simulink model "Friction_Estimation"  (R2024b)
settings: Solver=VariableStepAuto  StartTime=0.0  StopTime=45  RelTol=1e-3
InitFcn:
  | Init
values from neighbouring files (symbols this model uses):
  degs2rpm = 60/360    (= 0.166666666667)    [Init.m]    (also in ModelParams.m; load_params_inertial_case.m)
  delta_est = 1/sqrt(2)    [Init.m]    (also in code.m; main.m)
  Kd = Kp * Td    [Init.m]    (also in code.m; main.m)
  Ki = Kp / Ti    [Init.m]    (also in code.m; main.m)
  Kp = deltak * cos(deltaphi)    [Init.m]    (also in code.m = deltak*cos(deltaphi); main.m = deltak*cos(deltaphi))
  rpm2degs = 360/60    (= 6)    [Init.m]    (also in ModelParams.m; load_params_inertial_case.m)
  rpm2rads = 2*pi/60    (= 0.10471975512)    [Init.m]    (also in ModelParams.m; load_params_inertial_case.m)
  tl = 1/(3*wgc)    [Init.m]    (also in code.m = 1/cut_off; main.m = 1/cut_off)
  wc = 2*pi*20    (= 125.663706144)    [Init.m]    (also in code.m; main.m)
undefined symbols (not defined in the file or in its folder): gbox, mot, sens
libraries: simulink x2, SignalEditorBlockLib x1
settings Model: Creator=UTENTE041019  LastModifiedBy=lucag

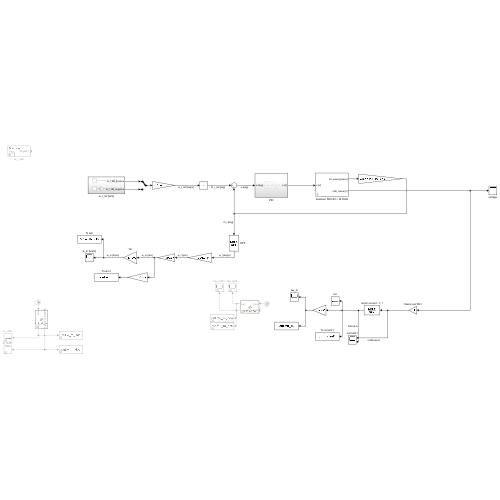
[thumbnail: Simulink's stored preview of the top-level diagram]
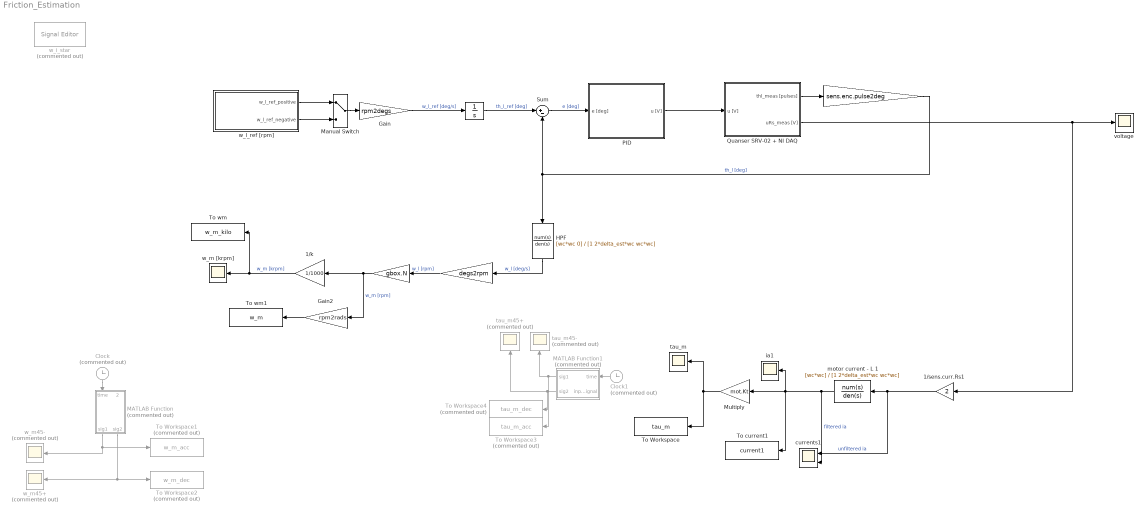
== system Friction_Estimation ==
  " " : Integrator
  "  " : Gain  Gain=sens.enc.pulse2deg
  "       " : Gain  Gain=degs2rpm
  "                  " : Gain  Gain=gbox.N
  1/k : Gain  Gain=1/1000
  1/sens.curr.Rs1 : Gain  Gain=2
  Clock : Clock  Commented=on
  Clock1 : Clock  Commented=on
  Gain : Gain  Gain=rpm2degs
  Gain2 : Gain  Gain=rpm2rads
  HPF : TransferFcn  Numerator=[wc*wc 0]  Denominator=[1 2*delta_est*wc wc*wc]
  MATLAB Function : MATLAB Function  Commented=on  TreatAsAtomicUnit=on
  MATLAB Function1 : MATLAB Function  Commented=on  TreatAsAtomicUnit=on
  Manual Switch : ManualSwitch
  Multiply : Gain  Gain=mot.Kt
  PID : Subsystem
  Quanser SRV-02 + NI DAQ : Subsystem  mask(Quanser SRV-02 (with inertial load) + NI DAQ){Ts=0.001, fricType=Coulomb + viscous}
      mask prompts: Ts "NI DAQ Sample Time:"; fricType "Friction model"
      mask help: Quanser SRV-02 (with inertial load) + NI DAQ model.
      mask init:
      | %%  Sensors data
      | 
      | %   shunt resistor
      | sens.curr.Rs = 0.5;                         %   resistance [Ohm]   
      | sens.curr.uRs_std = 0.01;                   %   voltage noise standard dev [V]                           
      | sens.curr.uRs_var = sens.curr.uRs_std^2;	%   voltage noise variance [V^2]
      | 
      | %   Hewlett-Packard HEDS-5540#A06 optical encoder
      | sens.enc.ppr = 500*4;                       %   pulses per rotation
      | sens.enc.pulse2deg = 360/sens.enc.ppr;      %   [pulses] -> [deg]
      | sens.enc.pulse2rad = 2*pi/sens.enc.ppr;     %   [pulses] -> [rad]
      | sens.enc.deg2pulse = sens.enc.ppr/360;      %   [deg] -> [pulses]
      | sens.enc.rad2pulse = sens.enc.ppr/2/pi;     %   [rad] -> [pulses]
      | 
      | 
      | %%  Data acquisition board (daq) data
      | 
      | %   NI PCI-6221 DAC data
      | daq.dac.bits = 16;                                  %   resolution (bits)
      | daq.dac.fs   = 10;                                  %   full scale 
      | daq.dac.q    = 2*daq.dac.fs/(2^daq.dac.bits-1);     %	quantization
      | 
      | %   NI PCI-6221 ADC data
      | daq.adc.bits = 16;                                  %   resolution (bits)
      | daq.adc.fs   = 10;                                  %   full scale (as set in SLDRT Analog Input block)
      | daq.adc.q    = 2*daq.adc.fs/(2^daq.adc.bits-1);     %   quantization
      mask Help:
      | Riccardo Antonello (antonello@dei.unipd.it)
      | 
      | April 24, 2020
      | 
      | Dept. of Information Engineering, University of Padova
      mask TypeOptions fricType: Coulomb + viscous | Karnopp
  Sum : Sum  Inputs=|+-
  To Workspace : ToWorkspace  VariableName=tau_m  SaveFormat=Structure With Time  SampleTime=-1
  To Workspace1 : ToWorkspace  Commented=on  VariableName=w_m_acc  SaveFormat=Structure With Time  SampleTime=-1
  To Workspace2 : ToWorkspace  Commented=on  VariableName=w_m_dec  SaveFormat=Structure With Time  SampleTime=-1
  To Workspace3 : ToWorkspace  Commented=on  VariableName=tau_m_acc  SaveFormat=Structure With Time  SampleTime=-1
  To Workspace4 : ToWorkspace  Commented=on  VariableName=tau_m_dec  SaveFormat=Structure With Time  SampleTime=-1
  To current1 : ToWorkspace  VariableName=current1  SaveFormat=Structure With Time  SampleTime=-1
  To wm : ToWorkspace  VariableName=w_m_kilo  SaveFormat=Structure With Time  SampleTime=-1
  To wm1 : ToWorkspace  VariableName=w_m  SaveFormat=Structure With Time  SampleTime=-1
  currents1 : Scope  NumInputPorts=2
  ia1 : Scope
  motor current - L 1 : TransferFcn  Numerator=[wc*wc]  Denominator=[1 2*delta_est*wc wc*wc]
  tau_m : Scope
  tau_m45+ : Scope  Commented=on
  tau_m45- : Scope  Commented=on
  voltage : Scope
  w_i_star : SignalEditorBlockLib/Signal Editor  Commented=on  FileName=untitled.mat  ActiveScenario=Scenario  ActiveSignal=Signal 1  IsBus=off  OutputBusObjectStr=Bus: BusObject  SampleTime=0  Interpolate=off  ZeroCross=off  OutputAfterFinalValue=Setting to zero  Unit=inherit  PreserveSignalName=on  ApplySigPropsToAllScenarios=on  ApplySigPropsToAllSignals=off
  w_l_ref [rpm] : Subsystem
  w_m [krpm] : Scope
  w_m45+ : Scope  Commented=on
  w_m45- : Scope  Commented=on
  wires:
  Sum/1 -> PID/1(e [deg])  "e [deg]"
  Quanser SRV-02 + NI DAQ/1(thl_meas [pulses]) -> "  "/1
  PID/1(u [V]) -> Quanser SRV-02 + NI DAQ/1(u [V])
  " "/1 -> Sum/1  "th_l_ref [deg]"
  "  "/1 -> HPF/1, Sum/2  "th_l [deg]"
  Quanser SRV-02 + NI DAQ/2(uRs_meas [V]) -> voltage/1, 1/sens.curr.Rs1/1
  1/sens.curr.Rs1/1 -> currents1/1, motor current - L 1/1  "unfiltered ia"
  motor current - L 1/1 -> currents1/2, ia1/1, Multiply/1, To current1/1  "filtered ia"
  HPF/1 -> "       "/1  "w_l [deg/s]"
  "       "/1 -> "                  "/1  "w_l [rpm]"
  "                  "/1 -> Gain2/1, 1/k/1  "w_m [rpm]"
  1/k/1 -> To wm/1, w_m [krpm]/1  "w_m [krpm]"
  Gain/1 -> " "/1  "w_l_ref [deg/s]"
  Clock/1 -> MATLAB Function/1(time)
  MATLAB Function/1(sig1) -> w_m45-/1, To Workspace1/1
  MATLAB Function/2(sig2) -> w_m45+/1, To Workspace2/1
  MATLAB Function1/2(sig2) -> tau_m45+/1, To Workspace4/1
  Clock1/1 -> MATLAB Function1/1(time)
  Multiply/1 -> tau_m/1, To Workspace/1
  MATLAB Function1/1(sig1) -> To Workspace3/1, tau_m45-/1
  w_l_ref [rpm]/1(w_l_ref_positive) -> Manual Switch/1
  w_l_ref [rpm]/2(w_l_ref_negative) -> Manual Switch/2
  Manual Switch/1 -> Gain/1
  Gain2/1 -> To wm1/1

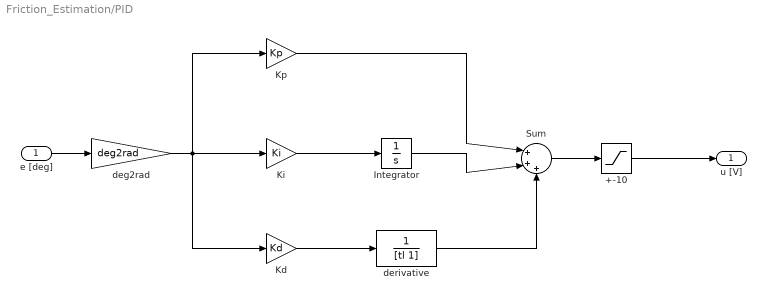
== system Friction_Estimation/PID ==
  e [deg] : Inport
  +-10 : Saturate  UpperLimit=10  LowerLimit=-10
  Integrator : Integrator
  Kd : Gain  Gain=Kd
  Ki : Gain  Gain=Ki
  Kp : Gain  Gain=Kp
  Sum : Sum  Inputs=|+++
  deg2rad : Gain  Gain=deg2rad
  derivative : TransferFcn  Denominator=[tl 1]
  u [V] : Outport
  wires:
  e [deg]/1 -> deg2rad/1
  deg2rad/1 -> Kd/1, Kp/1, Ki/1
  Ki/1 -> Integrator/1
  Kp/1 -> Sum/1
  Integrator/1 -> Sum/2
  Kd/1 -> derivative/1
  derivative/1 -> Sum/3
  Sum/1 -> +-10/1
  +-10/1 -> u [V]/1

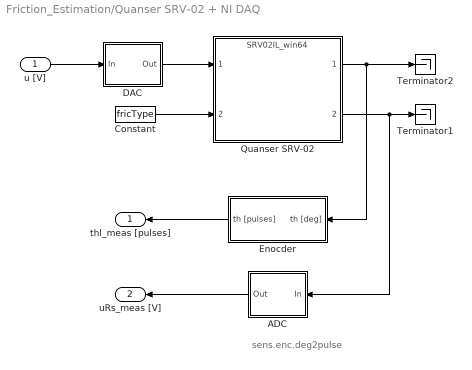
== system Friction_Estimation/Quanser SRV-02 + NI DAQ ==
  note: sens.enc.deg2pulse
  u [V] : Inport
  ADC : Subsystem
  Constant : Constant  Value=fricType
  DAC : Subsystem
  Enocder : Subsystem
  Quanser SRV-02 : ModelReference  ModelNameDialog=SRV02IL_win64.slxp  ModelReferenceVersion=1.44  CopyOfModelProtected=on
  Terminator1 : Terminator
  Terminator2 : Terminator
  thl_meas [pulses] : Outport
  uRs_meas [V] : Outport  Port=2
  wires:
  Enocder/1(th [pulses]) -> thl_meas [pulses]/1
  ADC/1(Out) -> uRs_meas [V]/1
  DAC/1(Out) -> Quanser SRV-02/1
  Quanser SRV-02/2 -> ADC/1(In), Terminator1/1
  u [V]/1 -> DAC/1(In)
  Quanser SRV-02/1 -> Enocder/1(th [deg]), Terminator2/1
  Constant/1 -> Quanser SRV-02/2

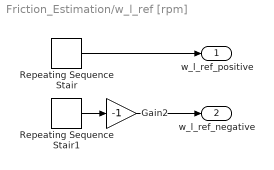
== system Friction_Estimation/w_l_ref [rpm] ==
  Gain2 : Gain  Gain=-1
  Repeating Sequence Stair : simulink/Sources/Repeating Sequence Stair  OutValues=[50 100 150 200 250 300 350 400 450 450].'  tsamp=5  OutMin=[]  OutMax=[]  OutDataTypeStr=double  OutputDataTypeScalingMode=double  OutDataType=fixdt(0,8)  ConRadixGroup=Best Precision: Vector-wise  OutScaling=2^-12
  Repeating Sequence Stair1 : simulink/Sources/Repeating Sequence Stair  OutValues=[50 100 150 200 250 300 350 400 450 450].'  tsamp=5  OutMin=[]  OutMax=[]  OutDataTypeStr=double  OutputDataTypeScalingMode=double  OutDataType=fixdt(0,8)  ConRadixGroup=Best Precision: Vector-wise  OutScaling=2^-12
  w_l_ref_positive : Outport
  w_l_ref_negative : Outport  Port=2
  wires:
  Repeating Sequence Stair1/1 -> Gain2/1
  Gain2/1 -> w_l_ref_negative/1
  Repeating Sequence Stair/1 -> w_l_ref_positive/1

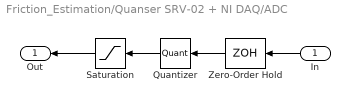
== system Friction_Estimation/Quanser SRV-02 + NI DAQ/ADC ==
  In : Inport
  Quantizer : Quantizer  QuantizationInterval=daq.adc.q
  Saturation : Saturate  UpperLimit=daq.adc.fs  LowerLimit=-daq.adc.fs
  Zero-Order Hold : ZeroOrderHold  SampleTime=Ts
  Out : Outport
  wires:
  Saturation/1 -> Out/1
  In/1 -> Zero-Order Hold/1
  Quantizer/1 -> Saturation/1
  Zero-Order Hold/1 -> Quantizer/1

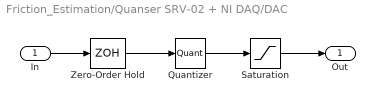
== system Friction_Estimation/Quanser SRV-02 + NI DAQ/DAC ==
  In : Inport
  Quantizer : Quantizer  QuantizationInterval=daq.dac.q
  Saturation : Saturate  UpperLimit=daq.dac.fs  LowerLimit=-daq.dac.fs
  Zero-Order Hold : ZeroOrderHold  SampleTime=Ts
  Out : Outport
  wires:
  Quantizer/1 -> Saturation/1
  In/1 -> Zero-Order Hold/1
  Zero-Order Hold/1 -> Quantizer/1
  Saturation/1 -> Out/1

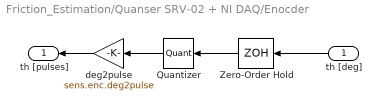
== system Friction_Estimation/Quanser SRV-02 + NI DAQ/Enocder ==
  th [deg] : Inport
  Quantizer : Quantizer  QuantizationInterval=sens.enc.pulse2deg
  Zero-Order Hold : ZeroOrderHold  SampleTime=Ts
  deg2pulse : Gain  Gain=sens.enc.deg2pulse
  th [pulses] : Outport
  wires:
  Quantizer/1 -> deg2pulse/1
  th [deg]/1 -> Zero-Order Hold/1
  Zero-Order Hold/1 -> Quantizer/1
  deg2pulse/1 -> th [pulses]/1

== matlab function Friction_Estimation/MATLAB Function ==
  data: time input; sig1 output; input_signal input; sig2 output
function [sig1, sig2] = split_signal(time, input_signal)
    if time <= 45
        sig1 = input_signal;
        sig2 = 0;
    else
        sig1 = 0;
        sig2 = input_signal;
    end
end

== matlab function Friction_Estimation/MATLAB Function1 ==
  data: time input; sig1 output; input_signal input; sig2 output
function [sig1, sig2] = split_signal(time, input_signal)
    if time <= 45
        sig1 = input_signal;
        sig2 = 0;
    else
        sig1 = 0;
        sig2 = input_signal;
    end
end
